simulink model "Signalflussplan4"  (R2026a)
settings: Solver=ode8  StopTime=20  FixedStep=Ta
values from neighbouring files (symbols this model uses):
  b1 = 2.39e6    (= 2390000)    [variablen.m]    (also in variablen2.m; variablen4.m)
  c_o = 36.5e6    (= 36500000)    [variablen.m]    (also in variablen2.m; variablen4.m)
  c_p = 75e6    (= 75000000)    [variablen.m]    (also in variablen2.m; variablen4.m)
  FN = F_N    (= 63000)    [variablen.m]    (also in variablen2.m; variablen4.m)
  i_vmax = 1    [variablen.m]    (also in variablen2.m; variablen4.m)
  K_L = 1    [variablen.m]    (also in variablen2.m; variablen4.m)
  K_sv = 0.796    [variablen.m]    (also in variablen2.m; variablen4.m)
  KI = 0.224    [variablen2.m]    (also in variablen4.m)
  KM = 1/63000    (= 1.5873015873e-05)    [variablen2.m]    (also in variablen4.m)
  m_g = m_k + m_p    (= 268.7)    [variablen.m]    (also in variablen2.m; variablen4.m)
  Ta = 0.015    [variablen2.m]    (also in variablen4.m)
libraries: slpidlib x3
settings Model: Creator=johannakruger
settings DataIOCC: ExternalInput=[0 0]  InitialState=[]  LoadExternalInput=on  LoadInitialState=on
settings OptimizationCC: BufferReuse=off
settings DebuggingCC: InitInArrayFormatMsg=none

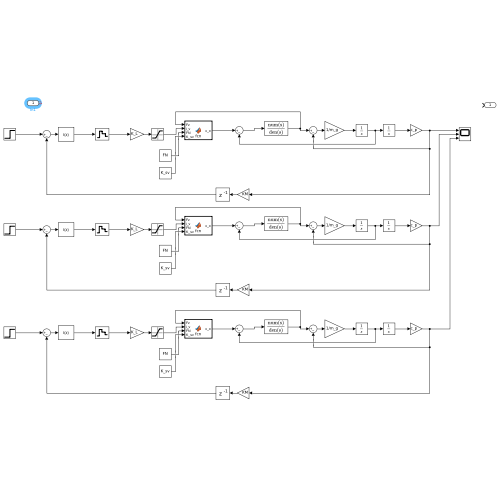
[thumbnail: Simulink's stored preview of the top-level diagram]
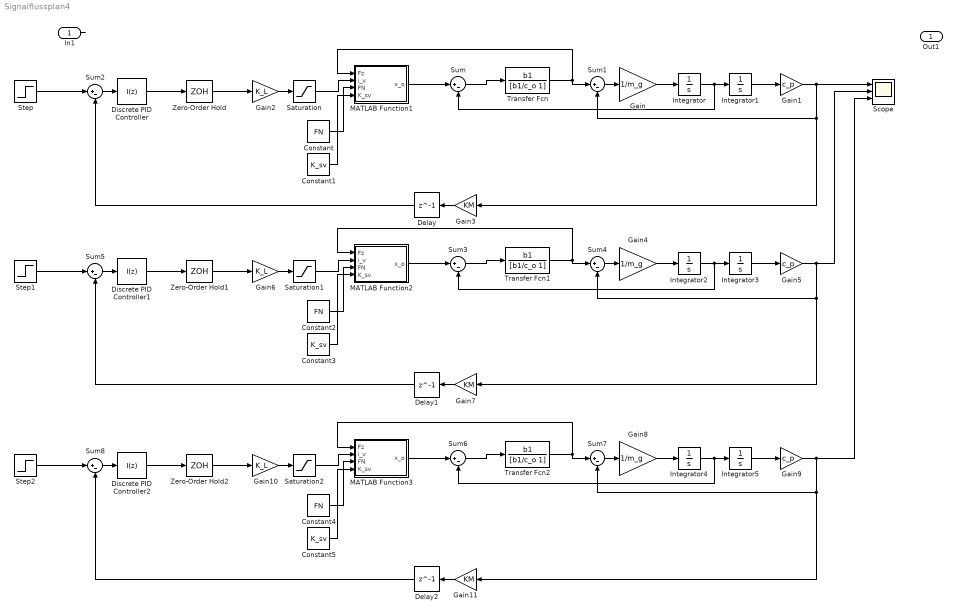
== system Signalflussplan4 ==
  In1 : Inport
  Constant : Constant  Value=FN
  Constant1 : Constant  Value=K_sv
  Constant2 : Constant  Value=FN
  Constant3 : Constant  Value=K_sv
  Constant4 : Constant  Value=FN
  Constant5 : Constant  Value=K_sv
  Delay : Delay  DelayLength=1  InitialCondition=0  SampleTime=Ta
  Delay1 : Delay  DelayLength=1  InitialCondition=0  SampleTime=Ta
  Delay2 : Delay  DelayLength=1  InitialCondition=0  SampleTime=Ta
  Discrete PID Controller : slpidlib/PID Controller  Controller=I  Form=Parallel  TimeDomain=Discrete-time  UseExternalTs=off  SampleTime=-1  IntegratorMethod=Forward Euler  FilterMethod=Forward Euler  ControllerParametersSource=internal  P=1  I=KI  UseKiTs=off  D=0  UseExternalDerivativeSource=off  N=100  UseFilter=on  TunerSelectOption=Transfer Function Based (PID Tuner App)  InitialConditionSource=internal  InitialConditionForIntegrator=0  InitialConditionForFilter=0  DifferentiatorICPrevScaledInput=0  ExternalReset=none  TrackingMode=off  Kt=1  LimitOutput=off  SatLimitsSource=internal  UpperSaturationLimit=inf  LowerSaturationLimit=-inf  LinearizeAsGain=off  AntiWindupMode=none  Kb=1  LimitIntegrator=off  UpperIntegratorSaturationLimit=inf  LowerIntegratorSaturationLimit=-inf  POutMin=[]  POutMax=[]  IOutMin=[]  IOutMax=[]  DOutMin=[]  DOutMax=[]  NOutMin=[]  NOutMax=[]  SumOutMin=[]  SumOutMax=[]  SaturationOutMin=[]  SaturationOutMax=[]  PParamMin=[]  PParamMax=[]  IParamMin=[]  IParamMax=[]  DParamMin=[]  DParamMax=[]  NParamMin=[]  NParamMax=[]  KbParamMin=[]  KbParamMax=[]  KtParamMin=[]  KtParamMax=[]  KbOutMin=[]  KbOutMax=[]  KtOutMin=[]  KtOutMax=[]  IntegratorOutMin=[]  IntegratorOutMax=[]  FilterOutMin=[]  FilterOutMax=[]  SumI1OutMin=[]  SumI1OutMax=[]  SumI2OutMin=[]  SumI2OutMax=[]  SumI3OutMin=[]  SumI3OutMax=[]  SumI4OutMin=[]  SumI4OutMax=[]  SumDOutMin=[]  SumDOutMax=[]  DifferentiatorOutMin=[]  DifferentiatorOutMax=[]  FilterDiffOutCoefMin=[]  FilterDiffOutCoefMax=[]  ReciprocalOutMin=[]  ReciprocalOutMax=[]  SumDenOutMin=[]  SumDenOutMax=[]  SumNumOutMin=[]  SumNumOutMax=[]  DivideOutMin=[]  DivideOutMax=[]  UdiffTsProdOutMin=[]  UdiffTsProdOutMax=[]  NTsProdOutMin=[]  NTsProdOutMax=[]  UintegralTsProdOutMin=[]  UintegralTsProdOutMax=[]  UngainTsProdOutMin=[]  UngainTsProdOutMax=[]  ClampingZeroOutDataTypeStr=Inherit: Inherit via back propagation  ClampingZeroOutMin=[]  ClampingZeroOutMax=[]  FilterDenConstantOutDataTypeStr=Inherit: Inherit via back propagation  FilterDenConstantOutMin=[]  FilterDenConstantOutMax=[]  PCopyOutDataTypeStr=Inherit: Inherit via back propagation  PCopyOutMin=[]  PCopyOutMax=[]  NCopyOutDataTypeStr=Inherit: Inherit via back propagation  NCopyOutMin=[]  NCopyOutMax=[]  IntegratorContinuousStateAttributes=''  IntegratorStateMustResolveToSignalObject=off  IntegratorRTWStateStorageClass=Auto  FilterContinuousStateAttributes=''  FilterStateMustResolveToSignalObject=off  FilterRTWStateStorageClass=Auto  ParallelPVariant=Disabled  IdealPVariant=Disabled  IVariant=InternalParameters  DVariant=Disabled  IntegratorVariant=Discrete  SatVariant=Disabled  AWVariant=Passthrough  PCopyVariant=Disabled  TRVariant=Disabled  FdbkBlocksVariant=Forward  IdealPFdbkVariant=Disabled  SatFdbkVariant=Disabled  DerivativeFilterVariant=Disabled  NVariant=Disabled  NCopyVariant=Disabled_SignalSpec  FilterICVariant=Disabled  IntegratorICVariant=InternalICs  ExternalResetVariant=Disabled  TRSumVariant=Passthrough  SumFdbkVariant=Disabled  SumVariant=Passthrough_I  TsampFilterVariant=InternalTs  TsampNgainVariant=Passthrough  TsampIntegralVariant=Disabled_SignalSpec  ExternalSaturationOutDataTypeStr=Inherit: Same as second input  DerivativeSourceVariant=Disabled  PreIntVariant=InternalPreInt
      settings: LibrarySourceBlock=simulink/Discrete/Discrete PID Controller
  Discrete PID Controller1 : slpidlib/PID Controller  Controller=I  Form=Parallel  TimeDomain=Discrete-time  UseExternalTs=off  SampleTime=-1  IntegratorMethod=Forward Euler  FilterMethod=Forward Euler  ControllerParametersSource=internal  P=1  I=KI  UseKiTs=off  D=0  UseExternalDerivativeSource=off  N=100  UseFilter=on  TunerSelectOption=Transfer Function Based (PID Tuner App)  InitialConditionSource=internal  InitialConditionForIntegrator=0  InitialConditionForFilter=0  DifferentiatorICPrevScaledInput=0  ExternalReset=none  TrackingMode=off  Kt=1  LimitOutput=off  SatLimitsSource=internal  UpperSaturationLimit=inf  LowerSaturationLimit=-inf  LinearizeAsGain=off  AntiWindupMode=none  Kb=1  LimitIntegrator=off  UpperIntegratorSaturationLimit=inf  LowerIntegratorSaturationLimit=-inf  POutMin=[]  POutMax=[]  IOutMin=[]  IOutMax=[]  DOutMin=[]  DOutMax=[]  NOutMin=[]  NOutMax=[]  SumOutMin=[]  SumOutMax=[]  SaturationOutMin=[]  SaturationOutMax=[]  PParamMin=[]  PParamMax=[]  IParamMin=[]  IParamMax=[]  DParamMin=[]  DParamMax=[]  NParamMin=[]  NParamMax=[]  KbParamMin=[]  KbParamMax=[]  KtParamMin=[]  KtParamMax=[]  KbOutMin=[]  KbOutMax=[]  KtOutMin=[]  KtOutMax=[]  IntegratorOutMin=[]  IntegratorOutMax=[]  FilterOutMin=[]  FilterOutMax=[]  SumI1OutMin=[]  SumI1OutMax=[]  SumI2OutMin=[]  SumI2OutMax=[]  SumI3OutMin=[]  SumI3OutMax=[]  SumI4OutMin=[]  SumI4OutMax=[]  SumDOutMin=[]  SumDOutMax=[]  DifferentiatorOutMin=[]  DifferentiatorOutMax=[]  FilterDiffOutCoefMin=[]  FilterDiffOutCoefMax=[]  ReciprocalOutMin=[]  ReciprocalOutMax=[]  SumDenOutMin=[]  SumDenOutMax=[]  SumNumOutMin=[]  SumNumOutMax=[]  DivideOutMin=[]  DivideOutMax=[]  UdiffTsProdOutMin=[]  UdiffTsProdOutMax=[]  NTsProdOutMin=[]  NTsProdOutMax=[]  UintegralTsProdOutMin=[]  UintegralTsProdOutMax=[]  UngainTsProdOutMin=[]  UngainTsProdOutMax=[]  ClampingZeroOutDataTypeStr=Inherit: Inherit via back propagation  ClampingZeroOutMin=[]  ClampingZeroOutMax=[]  FilterDenConstantOutDataTypeStr=Inherit: Inherit via back propagation  FilterDenConstantOutMin=[]  FilterDenConstantOutMax=[]  PCopyOutDataTypeStr=Inherit: Inherit via back propagation  PCopyOutMin=[]  PCopyOutMax=[]  NCopyOutDataTypeStr=Inherit: Inherit via back propagation  NCopyOutMin=[]  NCopyOutMax=[]  IntegratorContinuousStateAttributes=''  IntegratorStateMustResolveToSignalObject=off  IntegratorRTWStateStorageClass=Auto  FilterContinuousStateAttributes=''  FilterStateMustResolveToSignalObject=off  FilterRTWStateStorageClass=Auto  ParallelPVariant=Disabled  IdealPVariant=Disabled  IVariant=InternalParameters  DVariant=Disabled  IntegratorVariant=Discrete  SatVariant=Disabled  AWVariant=Passthrough  PCopyVariant=Disabled  TRVariant=Disabled  FdbkBlocksVariant=Forward  IdealPFdbkVariant=Disabled  SatFdbkVariant=Disabled  DerivativeFilterVariant=Disabled  NVariant=Disabled  NCopyVariant=Disabled_SignalSpec  FilterICVariant=Disabled  IntegratorICVariant=InternalICs  ExternalResetVariant=Disabled  TRSumVariant=Passthrough  SumFdbkVariant=Disabled  SumVariant=Passthrough_I  TsampFilterVariant=InternalTs  TsampNgainVariant=Passthrough  TsampIntegralVariant=Disabled_SignalSpec  ExternalSaturationOutDataTypeStr=Inherit: Same as second input  DerivativeSourceVariant=Disabled  PreIntVariant=InternalPreInt
      settings: LibrarySourceBlock=simulink/Discrete/Discrete PID Controller
  Discrete PID Controller2 : slpidlib/PID Controller  Controller=I  Form=Parallel  TimeDomain=Discrete-time  UseExternalTs=off  SampleTime=-1  IntegratorMethod=Forward Euler  FilterMethod=Forward Euler  ControllerParametersSource=internal  P=1  I=KI  UseKiTs=off  D=0  UseExternalDerivativeSource=off  N=100  UseFilter=on  TunerSelectOption=Transfer Function Based (PID Tuner App)  InitialConditionSource=internal  InitialConditionForIntegrator=0  InitialConditionForFilter=0  DifferentiatorICPrevScaledInput=0  ExternalReset=none  TrackingMode=off  Kt=1  LimitOutput=off  SatLimitsSource=internal  UpperSaturationLimit=inf  LowerSaturationLimit=-inf  LinearizeAsGain=off  AntiWindupMode=none  Kb=1  LimitIntegrator=off  UpperIntegratorSaturationLimit=inf  LowerIntegratorSaturationLimit=-inf  POutMin=[]  POutMax=[]  IOutMin=[]  IOutMax=[]  DOutMin=[]  DOutMax=[]  NOutMin=[]  NOutMax=[]  SumOutMin=[]  SumOutMax=[]  SaturationOutMin=[]  SaturationOutMax=[]  PParamMin=[]  PParamMax=[]  IParamMin=[]  IParamMax=[]  DParamMin=[]  DParamMax=[]  NParamMin=[]  NParamMax=[]  KbParamMin=[]  KbParamMax=[]  KtParamMin=[]  KtParamMax=[]  KbOutMin=[]  KbOutMax=[]  KtOutMin=[]  KtOutMax=[]  IntegratorOutMin=[]  IntegratorOutMax=[]  FilterOutMin=[]  FilterOutMax=[]  SumI1OutMin=[]  SumI1OutMax=[]  SumI2OutMin=[]  SumI2OutMax=[]  SumI3OutMin=[]  SumI3OutMax=[]  SumI4OutMin=[]  SumI4OutMax=[]  SumDOutMin=[]  SumDOutMax=[]  DifferentiatorOutMin=[]  DifferentiatorOutMax=[]  FilterDiffOutCoefMin=[]  FilterDiffOutCoefMax=[]  ReciprocalOutMin=[]  ReciprocalOutMax=[]  SumDenOutMin=[]  SumDenOutMax=[]  SumNumOutMin=[]  SumNumOutMax=[]  DivideOutMin=[]  DivideOutMax=[]  UdiffTsProdOutMin=[]  UdiffTsProdOutMax=[]  NTsProdOutMin=[]  NTsProdOutMax=[]  UintegralTsProdOutMin=[]  UintegralTsProdOutMax=[]  UngainTsProdOutMin=[]  UngainTsProdOutMax=[]  ClampingZeroOutDataTypeStr=Inherit: Inherit via back propagation  ClampingZeroOutMin=[]  ClampingZeroOutMax=[]  FilterDenConstantOutDataTypeStr=Inherit: Inherit via back propagation  FilterDenConstantOutMin=[]  FilterDenConstantOutMax=[]  PCopyOutDataTypeStr=Inherit: Inherit via back propagation  PCopyOutMin=[]  PCopyOutMax=[]  NCopyOutDataTypeStr=Inherit: Inherit via back propagation  NCopyOutMin=[]  NCopyOutMax=[]  IntegratorContinuousStateAttributes=''  IntegratorStateMustResolveToSignalObject=off  IntegratorRTWStateStorageClass=Auto  FilterContinuousStateAttributes=''  FilterStateMustResolveToSignalObject=off  FilterRTWStateStorageClass=Auto  ParallelPVariant=Disabled  IdealPVariant=Disabled  IVariant=InternalParameters  DVariant=Disabled  IntegratorVariant=Discrete  SatVariant=Disabled  AWVariant=Passthrough  PCopyVariant=Disabled  TRVariant=Disabled  FdbkBlocksVariant=Forward  IdealPFdbkVariant=Disabled  SatFdbkVariant=Disabled  DerivativeFilterVariant=Disabled  NVariant=Disabled  NCopyVariant=Disabled_SignalSpec  FilterICVariant=Disabled  IntegratorICVariant=InternalICs  ExternalResetVariant=Disabled  TRSumVariant=Passthrough  SumFdbkVariant=Disabled  SumVariant=Passthrough_I  TsampFilterVariant=InternalTs  TsampNgainVariant=Passthrough  TsampIntegralVariant=Disabled_SignalSpec  ExternalSaturationOutDataTypeStr=Inherit: Same as second input  DerivativeSourceVariant=Disabled  PreIntVariant=InternalPreInt
      settings: LibrarySourceBlock=simulink/Discrete/Discrete PID Controller
  Gain : Gain  Gain=1/m_g
  Gain1 : Gain  Gain=c_p
  Gain10 : Gain  Gain=K_L
  Gain11 : Gain  Gain=KM
  Gain2 : Gain  Gain=K_L
  Gain3 : Gain  Gain=KM
  Gain4 : Gain  Gain=1/m_g
  Gain5 : Gain  Gain=c_p
  Gain6 : Gain  Gain=K_L
  Gain7 : Gain  Gain=KM
  Gain8 : Gain  Gain=1/m_g
  Gain9 : Gain  Gain=c_p
  Integrator{,1..5} (6 alike) : Integrator
  MATLAB Function1 : MATLAB Function  TreatAsAtomicUnit=on
  MATLAB Function2 : MATLAB Function  TreatAsAtomicUnit=on
  MATLAB Function3 : MATLAB Function  TreatAsAtomicUnit=on
  Saturation : Saturate  UpperLimit=i_vmax  LowerLimit=-i_vmax
  Saturation1 : Saturate  UpperLimit=i_vmax  LowerLimit=-i_vmax
  Saturation2 : Saturate  UpperLimit=i_vmax  LowerLimit=-i_vmax
  Scope : Scope  NumInputPorts=3
      settings: ActiveDisplayYMinimum=-12913.53020978619  ActiveDisplayYMaximum=63663.363528997506
  Step : Step  FinalValue=0.1  SampleTime=0
  Step1 : Step  FinalValue=0.5  SampleTime=0
  Step2 : Step  FinalValue=0.8  SampleTime=0
  Sum{,1..8} (9 alike) : Sum  Inputs=|+-
  Transfer Fcn : TransferFcn  Numerator=b1  Denominator=[b1/c_o 1]
  Transfer Fcn1 : TransferFcn  Numerator=b1  Denominator=[b1/c_o 1]
  Transfer Fcn2 : TransferFcn  Numerator=b1  Denominator=[b1/c_o 1]
  Zero-Order Hold : ZeroOrderHold  SampleTime=Ta
  Zero-Order Hold1 : ZeroOrderHold  SampleTime=Ta
  Zero-Order Hold2 : ZeroOrderHold  SampleTime=Ta
  Out1 : Outport
  wires:
  Saturation/1 -> MATLAB Function1/2(i_v)
  Gain/1 -> Integrator/1
  Integrator1/1 -> Gain1/1
  MATLAB Function1/1(x_o) -> Sum/1
  Sum/1 -> Transfer Fcn/1
  Integrator/1 -> Sum/2, Integrator1/1
  Sum1/1 -> Gain/1
  Gain1/1 -> Gain3/1, Sum1/2, Scope/1
  Transfer Fcn/1 -> Sum1/1, MATLAB Function1/1(Fz)
  Constant/1 -> MATLAB Function1/3(FN)
  Constant1/1 -> MATLAB Function1/4(K_sv)
  Gain2/1 -> Saturation/1
  In1/1 -> ?
  Step/1 -> Sum2/1
  Discrete PID Controller/1 -> Zero-Order Hold/1
  Zero-Order Hold/1 -> Gain2/1
  Sum2/1 -> Discrete PID Controller/1
  Gain3/1 -> Delay/1
  Delay/1 -> Sum2/2
  Sum3/1 -> Transfer Fcn1/1
  Constant2/1 -> MATLAB Function2/3(FN)
  Gain5/1 -> Gain7/1, Sum4/2, Scope/2
  Gain6/1 -> Saturation1/1
  Gain7/1 -> Delay1/1
  Step1/1 -> Sum5/1
  Integrator2/1 -> Sum3/2, Integrator3/1
  Zero-Order Hold1/1 -> Gain6/1
  Sum4/1 -> Gain4/1
  MATLAB Function2/1(x_o) -> Sum3/1
  Transfer Fcn1/1 -> Sum4/1, MATLAB Function2/1(Fz)
  Saturation1/1 -> MATLAB Function2/2(i_v)
  Integrator3/1 -> Gain5/1
  Sum5/1 -> Discrete PID Controller1/1
  Discrete PID Controller1/1 -> Zero-Order Hold1/1
  Constant3/1 -> MATLAB Function2/4(K_sv)
  Gain4/1 -> Integrator2/1
  Delay1/1 -> Sum5/2
  Saturation2/1 -> MATLAB Function3/2(i_v)
  Delay2/1 -> Sum8/2
  Step2/1 -> Sum8/1
  Discrete PID Controller2/1 -> Zero-Order Hold2/1
  Gain10/1 -> Saturation2/1
  Gain9/1 -> Gain11/1, Sum7/2, Scope/3
  Gain11/1 -> Delay2/1
  Constant4/1 -> MATLAB Function3/3(FN)
  Sum8/1 -> Discrete PID Controller2/1
  Sum6/1 -> Transfer Fcn2/1
  Integrator4/1 -> Sum6/2, Integrator5/1
  Zero-Order Hold2/1 -> Gain10/1
  Sum7/1 -> Gain8/1
  Constant5/1 -> MATLAB Function3/4(K_sv)
  MATLAB Function3/1(x_o) -> Sum6/1
  Transfer Fcn2/1 -> Sum7/1, MATLAB Function3/1(Fz)
  Integrator5/1 -> Gain9/1
  Gain8/1 -> Integrator4/1

== matlab function Signalflussplan4/MATLAB Function1 ==
  data: Fz input; i_v input; x_o output; FN input; K_sv input
function x_o = fcn(Fz, i_v, FN, K_sv)

A = 1 - Fz/FN * sign(i_v);

if A <= 0
    x_o = 0;
else
    x_o = i_v * K_sv * sqrt(A);
end

== matlab function Signalflussplan4/MATLAB Function2 ==
  data: Fz input; i_v input; x_o output; FN input; K_sv input
function x_o = fcn(Fz, i_v, FN, K_sv)

A = 1 - Fz/FN * sign(i_v);

if A <= 0
    x_o = 0;
else
    x_o = i_v * K_sv * sqrt(A);
end

== matlab function Signalflussplan4/MATLAB Function3 ==
  data: Fz input; i_v input; x_o output; FN input; K_sv input
function x_o = fcn(Fz, i_v, FN, K_sv)

A = 1 - Fz/FN * sign(i_v);

if A <= 0
    x_o = 0;
else
    x_o = i_v * K_sv * sqrt(A);
end
